simulink model "Foor_loop_parallel_func"  (R2021b)
settings: Solver=FixedStepAuto  StartTime=0.0  StopTime=101  FixedStep=50  RelTol=1e-3
settings Model: Creator=vgaggero  LastModifiedBy=vgaggero

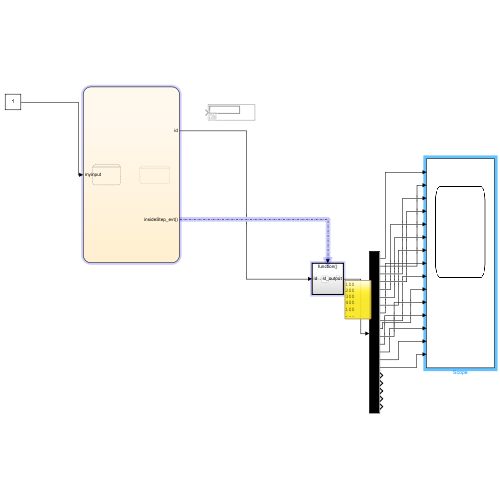
[thumbnail: Simulink's stored preview of the top-level diagram]
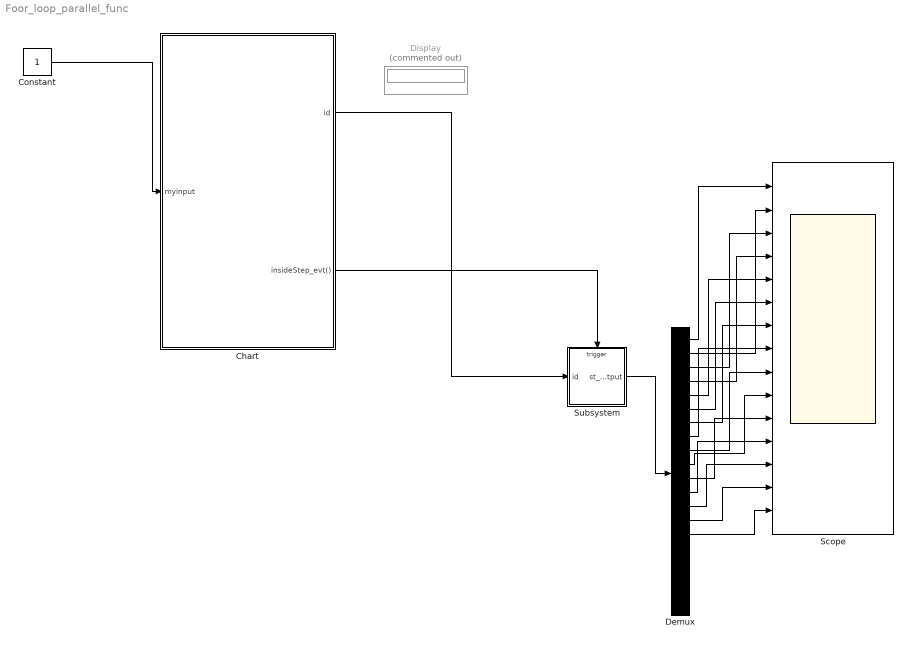
== system Foor_loop_parallel_func ==
  Chart : Stateflow chart  TreatAsAtomicUnit=on
  Constant : Constant  OutDataTypeStr=int32
  Demux : Demux  Outputs=20
  Display : Display  Commented=on
  Scope : Scope  NumInputPorts=15
  Subsystem : Subsystem
  wires:
  Constant/1 -> Chart/1(myinput)
  Chart/2(insideStep_evt()) -> Subsystem/Trigger
  Subsystem/1(st_output) -> Demux/1
  Chart/1(id) -> Subsystem/1(id)
  Demux/1 -> Scope/1
  Demux/2 -> Scope/2
  Demux/3 -> Scope/3
  Demux/4 -> Scope/4
  Demux/5 -> Scope/5
  Demux/6 -> Scope/6
  Demux/7 -> Scope/7
  Demux/8 -> Scope/8
  Demux/9 -> Scope/9
  Demux/10 -> Scope/10
  Demux/11 -> Scope/11
  Demux/12 -> Scope/12
  Demux/13 -> Scope/13
  Demux/14 -> Scope/14
  Demux/15 -> Scope/15

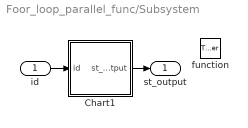
== system Foor_loop_parallel_func/Subsystem ==
  id : Inport
  function : TriggerPort  TriggerType=function-call  VariantControl=(inherit)
  Chart1 : Stateflow chart  TreatAsAtomicUnit=on
  st_output : Outport
  wires:
  Chart1/1(st_output) -> st_output/1
  id/1 -> Chart1/1(id)

== stateflow chart Foor_loop_parallel_func/Subsystem/Chart1 ==
  state stato_1
    entry:
    st_output(id)=100;
  state stato_2
    entry:
    st_output(id)=200;
  state stato_4
    entry:
    st_output(id)=400;
  state stato_3
    entry:
    st_output(id)=300;
  (default) -> stato_1
  stato_1 -> stato_2
  stato_4 -> stato_1
  stato_2 -> stato_3
  stato_3 -> stato_4
  data: st_output output int32 size=20; id input int32 size=1

== stateflow chart Foor_loop_parallel_func/Chart ==
  state for_loop [parallel]
    settings: executionOrder=1
    (default) -> (junction 5)
    (junction 5) -> (junction 7) : {index=1}
    (junction 7) -> (junction 9) [order 1] : [index<7]
    (junction 9) -> (junction 11) : {id=id+1;send(insideStep_evt);}
    (junction 11) -> (junction 7) : {index = index + 1}
    (junction 7) -> (junction 19) [order 2]
  state my_state_machine [parallel] [commented out]
    state Home [commented out]
      entry:
      output=100;
      du:
      output=index;
    (default) -> Home [commented out]
    Home -> Home [commented out] : [insideStep_evt]{output=output+1;}
  data: myinput input int32 size=1; index local int32 size=1; id output int32 size=1 =int32(0); data local int32 =int32(0)
  events: insideStep_evt output FUNCTION_CALL_EVENT
